simulink model "s2"  (R2016b)
settings: Solver=VariableStepAuto  StartTime=0.0  StopTime=10.0  RelTol=1e-3
settings Model: Creator=fabia  LastModifiedBy=fabia

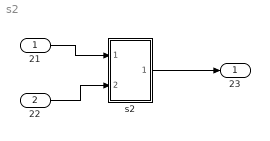
== system s2 ==
  21 : Inport
  22 : Inport  Port=2
  s2 : Subsystem
  23 : Outport
  wires:
  21/1 -> s2/1(In1)
  22/1 -> s2/2(In2)
  s2/1(Out1) -> 23/1

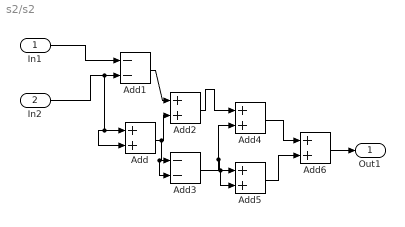
== system s2/s2 ==
  In1 : Inport
  In2 : Inport  Port=2
  Add{,2,4..6} (5 alike) : Sum
  Add1 : Sum  Inputs=--
  Add3 : Sum  Inputs=--
  Out1 : Outport
  wires:
  Add1/1 -> Add2/1
  In1/1 -> Add1/1
  In2/1 -> Add/2, Add/1, Add1/2
  Add/1 -> Add3/2, Add3/1, Add2/2
  Add2/1 -> Add4/1
  Add3/1 -> Add5/2, Add5/1, Add4/2
  Add6/1 -> Out1/1
  Add5/1 -> Add6/2
  Add4/1 -> Add6/1
